simulink model "Fdi_Device"  (R2020a)
settings: Solver=VariableStepAuto  StartTime=0.0  StopTime=10.0  RelTol=1e-3
undefined symbols (not defined in the file): fdiDevices, regs_z, T
libraries: PhdLibrary x2
settings Model: Creator=d13go  LastModifiedBy=d13go

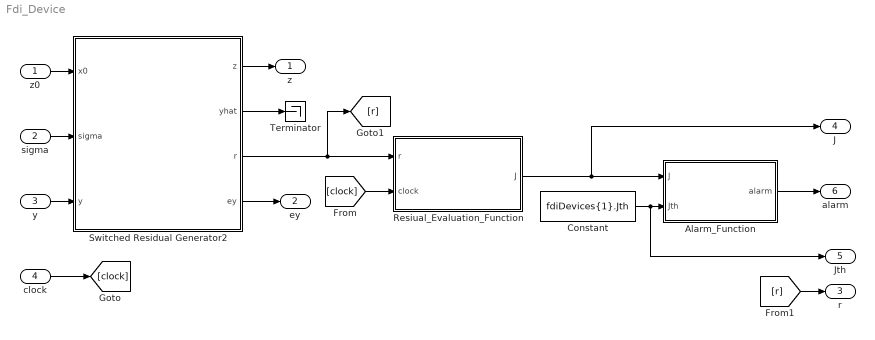
== system Fdi_Device ==
  z0 : Inport  PortDimensions=4
  sigma : Inport  Port=2
  y : Inport  Port=3  PortDimensions=3
  clock : Inport  Port=4
  Alarm_Function : Subsystem
  Constant : Constant  Value=fdiDevices{1}.Jth
  Resiual_Evaluation_Function : Subsystem
  Switched Residual Generator2 : Subsystem  AncestorBlock=PhdLibrary/Observers/Switched Residual Generator  mask(Boots State-Space model){reg_z=regs_z{1}}
      mask prompts: reg_z "Residual error generator (struct)"
      mask help: Boots State-Space model
      mask DialogControl DescTextVar Prompt: dxhat/dt = A(sigma)*xhat+B(sigma)*u + L(sigma)*(y-yhat)
      mask DialogControl Control2 Prompt: yhat = C(sigma)*xhat
      mask DialogControl Control3 Prompt: r = R(sigma)*(y-yhat)
      mask DialogControl Subsystem1 Prompt: Subsystem 1
      mask Display: disp('Switched Luenberger \n Residual Generator \n 2-Subsystems')
  Terminator : Terminator
  z : Outport
  ey : Outport  Port=2
  r : Outport  Port=3
  J : Outport  Port=4
  Jth : Outport  Port=5
  alarm : Outport  Port=6
  wires:
  Switched Residual Generator2/3(r) -> [r], Resiual_Evaluation_Function/1(r)
  Switched Residual Generator2/1(z) -> z/1
  Switched Residual Generator2/2(yhat) -> Terminator/1
  Resiual_Evaluation_Function/1(J) -> J/1, Alarm_Function/1(J)
  Constant/1 -> Jth/1, Alarm_Function/2(Jth)
  Switched Residual Generator2/4(ey) -> ey/1
  z0/1 -> Switched Residual Generator2/1(x0)
  sigma/1 -> Switched Residual Generator2/2(sigma)
  y/1 -> Switched Residual Generator2/3(y)
  clock/1 -> [clock]
  [clock] -> Resiual_Evaluation_Function/2(clock)
  Alarm_Function/1(alarm) -> alarm/1
  [r] -> r/1

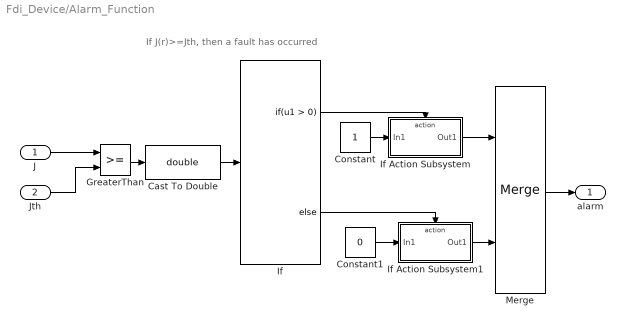
== system Fdi_Device/Alarm_Function ==
  note: If J(r)>=Jth, then a fault has occurred
  J : Inport
  Jth : Inport  Port=2
  Cast To Double : DataTypeConversion  OutDataTypeStr=double
  Constant : Constant
  Constant1 : Constant  Value=0
  GreaterThan : RelationalOperator  OutDataTypeStr=boolean  RndMeth=Simplest
  If : If
  If Action Subsystem : Subsystem  TreatAsAtomicUnit=on
  If Action Subsystem1 : Subsystem  TreatAsAtomicUnit=on
  Merge : Merge
  alarm : Outport
  wires:
  J/1 -> GreaterThan/1
  Jth/1 -> GreaterThan/2
  If/1 -> If Action Subsystem/Action
  Constant/1 -> If Action Subsystem/1(In1)
  If/2 -> If Action Subsystem1/Action
  Constant1/1 -> If Action Subsystem1/1(In1)
  If Action Subsystem/1(Out1) -> Merge/1
  If Action Subsystem1/1(Out1) -> Merge/2
  Merge/1 -> alarm/1
  GreaterThan/1 -> Cast To Double/1
  Cast To Double/1 -> If/1

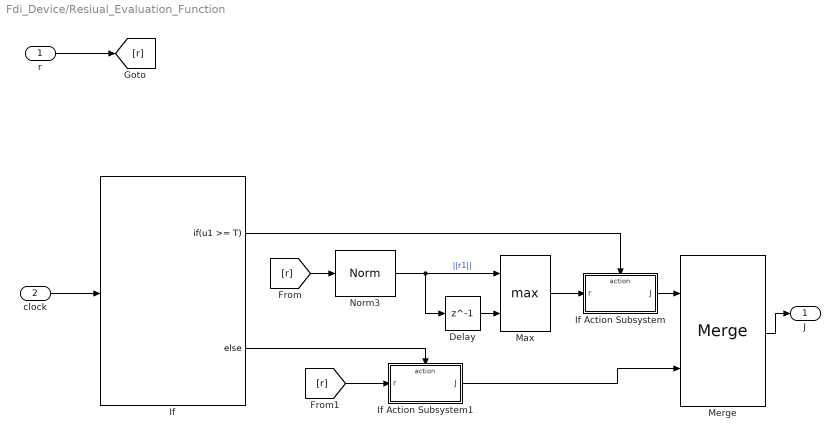
== system Fdi_Device/Resiual_Evaluation_Function ==
  r : Inport
  clock : Inport  Port=2
  Delay : Delay  DelayLength=1  SampleTime=T
  If : If  IfExpression=u1 >= T
  If Action Subsystem : Subsystem  TreatAsAtomicUnit=on
  If Action Subsystem1 : Subsystem  TreatAsAtomicUnit=on
  Max : MinMax  Function=max  Inputs=2
  Merge : Merge
  Norm3 : PhdLibrary/Norms/Norm
      settings: SourceProductName=Phd Diego
  J : Outport
  wires:
  clock/1 -> If/1
  If/1 -> If Action Subsystem/Action
  If/2 -> If Action Subsystem1/Action
  r/1 -> [r]
  [r] -> Norm3/1
  [r] -> If Action Subsystem1/1(r)
  If Action Subsystem/1(J) -> Merge/1
  If Action Subsystem1/1(J) -> Merge/2
  Merge/1 -> J/1
  Delay/1 -> Max/2
  Norm3/1 -> Max/1, Delay/1  "||r1||"
  Max/1 -> If Action Subsystem/1(r)

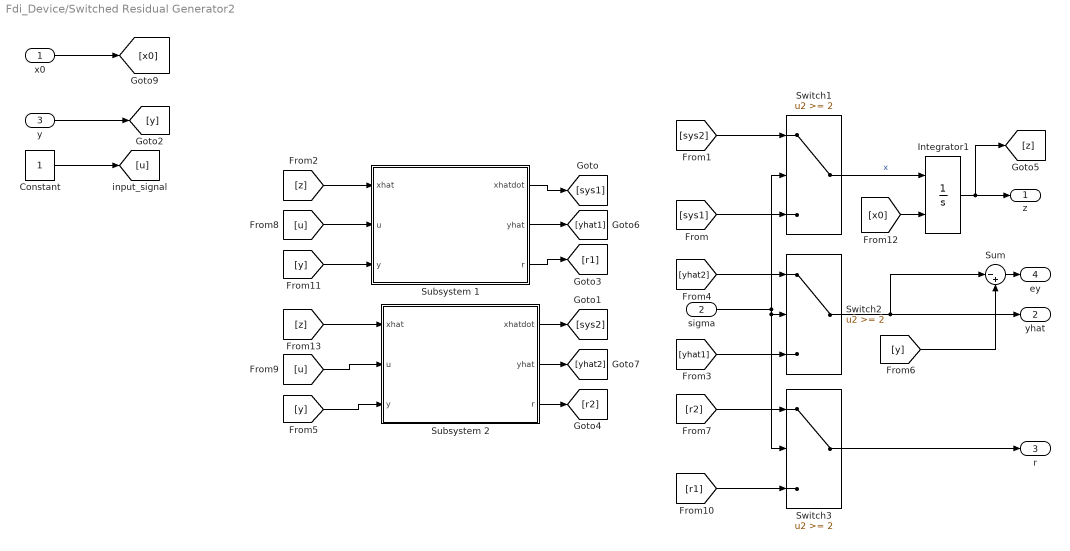
== system Fdi_Device/Switched Residual Generator2 ==
  x0 : Inport
  sigma : Inport  Port=2
  y : Inport  Port=3
  Constant : Constant
  Integrator1 : Integrator  InitialConditionSource=external  InitialCondition=[0; 0; 0;0]
  Subsystem 1 : Subsystem  mask{A=reg_z.Asigma{1}, B=reg_z.bsigma{1}, L=reg_z.Lsigma{1}, C=reg_z.Csigma{1}, R=reg_z.Rsigma{1}}
      mask prompts: A "Matrix A"; B "Matrix B"; L "Matrix L"; C "Matrix C"; R "Matrix R"
      mask DialogControl DescTextVar Prompt: dxhat/dt = A*xhat + B*u + L*(y-yhat)
      mask DialogControl Control2 Prompt: yhat = C*xhat
      mask Display: disp('Luenberger Residual \n Generator')
  Subsystem 2 : Subsystem  mask{A=reg_z.Asigma{2}, B=reg_z.bsigma{2}, L=reg_z.Lsigma{2}, C=reg_z.Csigma{2}, R=reg_z.Rsigma{2}}
      mask prompts: A "Matrix A"; B "Matrix B"; L "Matrix L"; C "Matrix C"; R "Matrix R"
      mask DialogControl DescTextVar Prompt: dxhat/dt = A*xhat + B*u + L*(y-yhat)
      mask DialogControl Control2 Prompt: yhat = C*xhat
      mask Display: disp('Luenberger Residual \n Generator')
  Sum : Sum  Inputs=|-+
  Switch1 : Switch  Threshold=2
  Switch2 : Switch  Threshold=2
  Switch3 : Switch  Threshold=2
  z : Outport
  yhat : Outport  Port=2
  r : Outport  Port=3
  ey : Outport  Port=4
  wires:
  [yhat2] -> Switch2/1
  [yhat1] -> Switch2/3
  [y] -> Sum/2
  Sum/1 -> ey/1
  y/1 -> [y]
  [y] -> Subsystem 2/3(y)
  Switch3/1 -> r/1
  Switch2/1 -> yhat/1, Sum/1
  [r1] -> Switch3/3
  [r2] -> Switch3/1
  Subsystem 2/2(yhat) -> [yhat2]
  Subsystem 1/2(yhat) -> [yhat1]
  Subsystem 2/3(r) -> [r2]
  Subsystem 1/3(r) -> [r1]
  Subsystem 2/1(xhatdot) -> [sys2]
  Subsystem 1/1(xhatdot) -> [sys1]
  x0/1 -> [x0]
  Switch1/1 -> Integrator1/1  "x"
  [sys1] -> Switch1/3
  [sys2] -> Switch1/1
  Integrator1/1 -> [z], z/1
  sigma/1 -> Switch1/2, Switch2/2, Switch3/2
  Constant/1 -> [u]
  [u] -> Subsystem 1/2(u)
  [u] -> Subsystem 2/2(u)
  [y] -> Subsystem 1/3(y)
  [z] -> Subsystem 1/1(xhat)
  [z] -> Subsystem 2/1(xhat)
  [x0] -> Integrator1/2

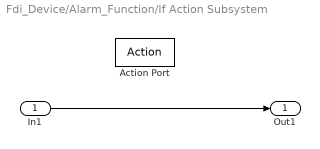
== system Fdi_Device/Alarm_Function/If Action Subsystem ==
  In1 : Inport
  Action Port : ActionPort  ActionPortLabel=if(u1 > 0)
  Out1 : Outport
  wires:
  In1/1 -> Out1/1

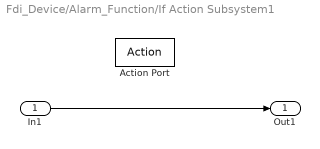
== system Fdi_Device/Alarm_Function/If Action Subsystem1 ==
  In1 : Inport
  Action Port : ActionPort  ActionPortLabel=else
  Out1 : Outport
  wires:
  In1/1 -> Out1/1

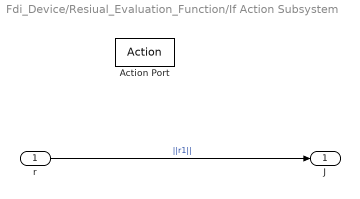
== system Fdi_Device/Resiual_Evaluation_Function/If Action Subsystem ==
  r : Inport
  Action Port : ActionPort  ActionPortLabel=if(u1 >= T)
  J : Outport
  wires:
  r/1 -> J/1  "||r1||"

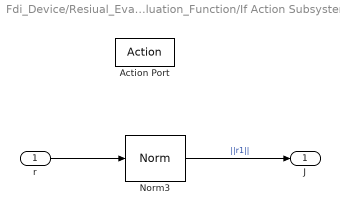
== system Fdi_Device/Resiual_Evaluation_Function/If Action Subsystem1 ==
  r : Inport
  Action Port : ActionPort  ActionPortLabel=else
  Norm3 : PhdLibrary/Norms/Norm
      settings: SourceProductName=Phd Diego
  J : Outport
  wires:
  r/1 -> Norm3/1
  Norm3/1 -> J/1  "||r1||"

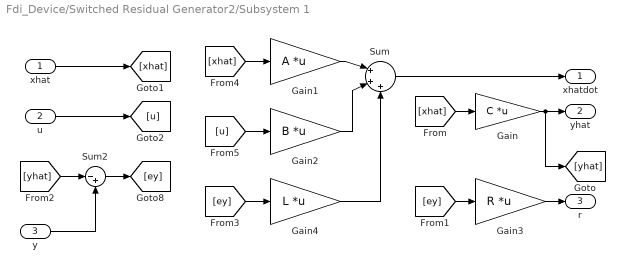
== system Fdi_Device/Switched Residual Generator2/Subsystem 1 ==
  xhat : Inport
  u : Inport  Port=2
  y : Inport  Port=3
  Gain : Gain  Gain=C  Multiplication=Matrix(K*u) (u vector)
  Gain1 : Gain  Gain=A  Multiplication=Matrix(K*u) (u vector)
  Gain2 : Gain  Gain=B  Multiplication=Matrix(K*u) (u vector)
  Gain3 : Gain  Gain=R  Multiplication=Matrix(K*u) (u vector)
  Gain4 : Gain  Gain=L  Multiplication=Matrix(K*u) (u vector)
  Sum : Sum  Inputs=|+++
  Sum2 : Sum  Inputs=|-+
  xhatdot : Outport
  yhat : Outport  Port=2
  r : Outport  Port=3
  wires:
  [ey] -> Gain4/1
  Gain4/1 -> Sum/3
  Gain2/1 -> Sum/2
  [u] -> Gain2/1
  Gain1/1 -> Sum/1
  [xhat] -> Gain1/1
  u/1 -> [u]
  Gain3/1 -> r/1
  [ey] -> Gain3/1
  [xhat] -> Gain/1
  xhat/1 -> [xhat]
  Gain/1 -> [yhat], yhat/1
  Sum/1 -> xhatdot/1
  y/1 -> Sum2/2
  [yhat] -> Sum2/1
  Sum2/1 -> [ey]

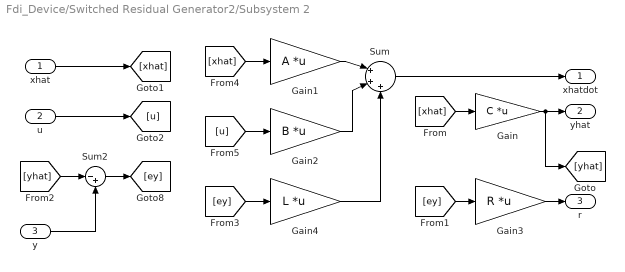
== system Fdi_Device/Switched Residual Generator2/Subsystem 2 ==
  xhat : Inport
  u : Inport  Port=2
  y : Inport  Port=3
  Gain : Gain  Gain=C  Multiplication=Matrix(K*u) (u vector)
  Gain1 : Gain  Gain=A  Multiplication=Matrix(K*u) (u vector)
  Gain2 : Gain  Gain=B  Multiplication=Matrix(K*u) (u vector)
  Gain3 : Gain  Gain=R  Multiplication=Matrix(K*u) (u vector)
  Gain4 : Gain  Gain=L  Multiplication=Matrix(K*u) (u vector)
  Sum : Sum  Inputs=|+++
  Sum2 : Sum  Inputs=|-+
  xhatdot : Outport
  yhat : Outport  Port=2
  r : Outport  Port=3
  wires:
  [ey] -> Gain4/1
  Gain4/1 -> Sum/3
  Gain2/1 -> Sum/2
  [u] -> Gain2/1
  Gain1/1 -> Sum/1
  [xhat] -> Gain1/1
  u/1 -> [u]
  Gain3/1 -> r/1
  [ey] -> Gain3/1
  [xhat] -> Gain/1
  xhat/1 -> [xhat]
  Gain/1 -> [yhat], yhat/1
  Sum/1 -> xhatdot/1
  y/1 -> Sum2/2
  [yhat] -> Sum2/1
  Sum2/1 -> [ey]
